simulink model "PDGravityCompensation"  (R2020b)
settings: Solver=VariableStepAuto  StartTime=0.0  StopTime=4  RelTol=1e-3
values from neighbouring files (symbols this model uses):
  he = u(4:9)    [Manipulator.m]    (also in params.m = zeros(6,1))
  Kd = diag([50 50 50])    [params.m]
  Kp = diag([700 700 700])    [params.m]
  qd = [0.3, 0.45, 0.2]    [params.m]
settings Model: Creator=andre  LastModifiedBy=filippo

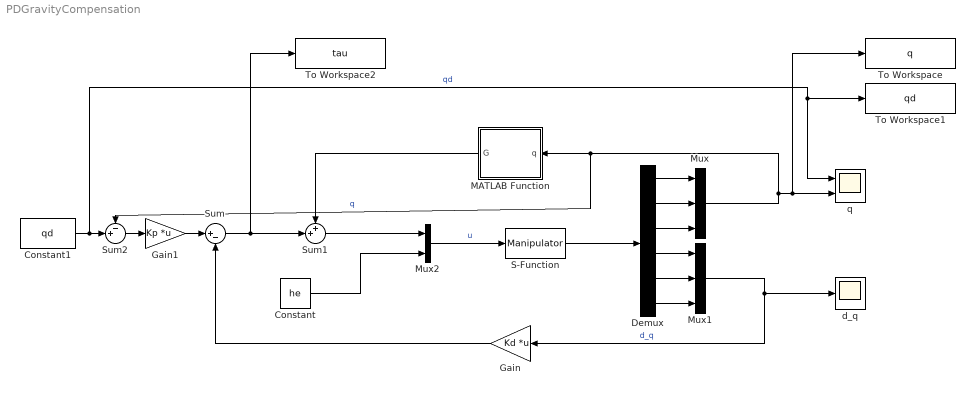
== system PDGravityCompensation ==
  Constant : Constant  Value=he
  Constant1 : Constant  Value=qd
  Demux : Demux  Outputs=6
  Gain : Gain  Gain=Kd  Multiplication=Matrix(K*u)
  Gain1 : Gain  Gain=Kp  Multiplication=Matrix(K*u)
  MATLAB Function : MATLAB Function  TreatAsAtomicUnit=on
  Mux : Mux  Inputs=3
  Mux1 : Mux  Inputs=3
  Mux2 : Mux  Inputs=2
  S-Function : S-Function  FunctionName=Manipulator  Parameters=param  SFunctionDeploymentMode=off  EnableBusSupport=off
  Sum : Sum  Inputs=|+-
  Sum1 : Sum  Inputs=++|
  Sum2 : Sum  Inputs=-+|
  To Workspace : ToWorkspace  VariableName=q  SaveFormat=Timeseries  SampleTime=-1
  To Workspace1 : ToWorkspace  VariableName=qd  SaveFormat=Timeseries  SampleTime=-1
  To Workspace2 : ToWorkspace  VariableName=tau  SaveFormat=Timeseries  SampleTime=-1
  d_q : Scope
  q : Scope  NumInputPorts=2
  wires:
  Sum/1 -> To Workspace2/1, Sum1/2
  Gain1/1 -> Sum/1
  MATLAB Function/1(G) -> Sum1/1
  S-Function/1 -> Demux/1
  Demux/3 -> Mux/3
  Demux/2 -> Mux/2
  Demux/1 -> Mux/1
  Demux/4 -> Mux1/1
  Demux/5 -> Mux1/2
  Demux/6 -> Mux1/3
  Mux/1 -> MATLAB Function/1(q), Sum2/1, To Workspace/1, q/2  "q"
  Constant/1 -> Mux2/2
  Sum1/1 -> Mux2/1
  Mux2/1 -> S-Function/1  "u"
  Gain/1 -> Sum/2
  Sum2/1 -> Gain1/1
  Constant1/1 -> To Workspace1/1, q/1, Sum2/2  "qd"
  Mux1/1 -> d_q/1, Gain/1  "d_q"

== matlab function PDGravityCompensation/MATLAB Function ==
  data: q input; G output; param parameter
function G = Gravity(q, param)
    t1 = q(1);
    d3 = q(3);

    g = param.g;
    l1 = param.l1;
    l3 = param.l3;
    m1 = param.m1;
    m2 = param.m2;
    m3 = param.m3;


    G = [ (g*cos(t1)*(2*d3*m3 + l1*m1 + 2*l1*m2 + 2*l1*m3 + l3*m3))/2;
                                                              0;
                                                   g*m3*sin(t1)];
end
